simulink model "sampleModel"  (R2021b)
settings: Solver=VariableStepAuto  StartTime=0.0  StopTime=10.0  RelTol=1e-3
settings Model: SimulationMode=accelerator  Creator=O  LastModifiedBy=wangzixuan

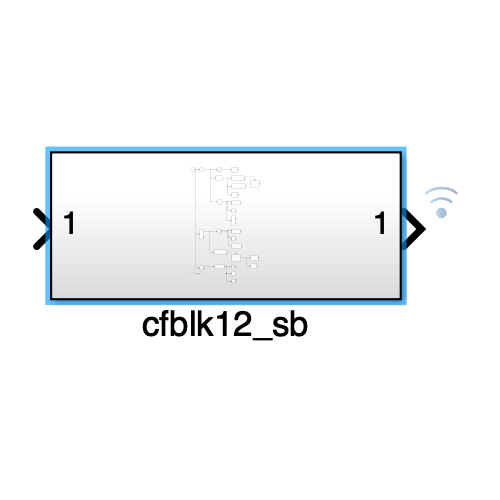
[thumbnail: Simulink's stored preview of the top-level diagram]
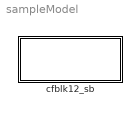
== system sampleModel ==
  cfblk12_sb : Subsystem

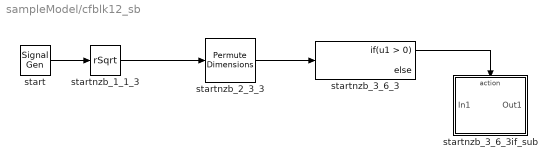
== system sampleModel/cfblk12_sb ==
  start : SignalGenerator  Units=rad/sec
  startnzb_1_1_3 : Sqrt  Operator=rSqrt  SaturateOnIntegerOverflow=on
  startnzb_2_3_3 : PermuteDimensions
  startnzb_3_6_3 : If
  startnzb_3_6_3if_sub : Subsystem  TreatAsAtomicUnit=on
  wires:
  startnzb_2_3_3/1 -> startnzb_3_6_3/1
  startnzb_1_1_3/1 -> startnzb_2_3_3/1
  start/1 -> startnzb_1_1_3/1
  startnzb_3_6_3/1 -> startnzb_3_6_3if_sub/Action

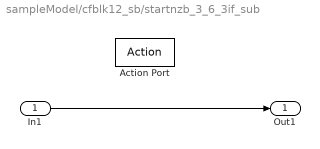
== system sampleModel/cfblk12_sb/startnzb_3_6_3if_sub ==
  In1 : Inport
  Action Port : ActionPort  ActionPortLabel=if(u1 > 0)
  Out1 : Outport
  wires:
  In1/1 -> Out1/1
